simulink model "arduino_write"  (R2021a)
settings: Solver=FixedStepAuto  StartTime=0.0  StopTime=1  FixedStep=0.001  RelTol=1e-3
libraries: arduinolib x1
settings Model: Creator=carol  LastModifiedBy=carol

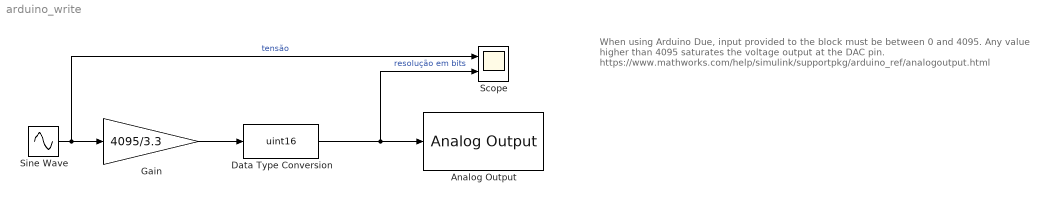
== system arduino_write ==
  note: When using Arduino Due, input provided to the block must be between 0 and 4095. Any value higher than 4095 saturates the voltage output at the DAC pin.
      |
      | https://www.mathworks.com/help/simulink/supportpkg/arduino_ref/analogoutput.html
  Analog Output : arduinolib/Analog Output  DACpin=DAC0  blockPlatform=arduino
      settings: SourceProductBaseCode=ARDUINO
  Data Type Conversion : DataTypeConversion  OutDataTypeStr=uint16
  Gain : Gain  Gain=4095/3.3
  Scope : Scope  NumInputPorts=2
  Sine Wave : Sin  Amplitude=1.5  Bias=1.5  Frequency=2*pi*1  SampleTime=0
  wires:
  Sine Wave/1 -> Gain/1, Scope/1  "tensão"
  Gain/1 -> Data Type Conversion/1
  Data Type Conversion/1 -> Scope/2, Analog Output/1  "resolução em bits"
